simulink model "simplequeu"  (R2013a)
settings: Solver=ode45  StartTime=0.0  StopTime=10.0  RelTol=1e-3
undefined symbols (not defined in the file or in its folder): des, gcbh
settings Model: Creator=daniel  LastModifiedBy=daniel

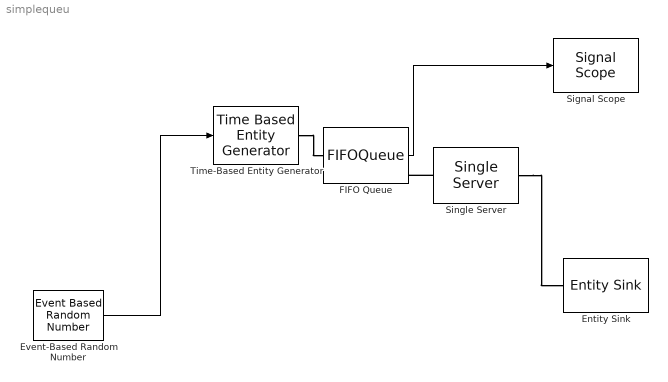
== system simplequeu ==
  Entity Sink : EntitySink  StatNumberArrived=on
  Event-Based Random Number : EventBasedRandomNumber  Distribution=Gaussian (normal)  meanNorm=90  stdNorm=3
  FIFO Queue : FIFOQueue  Capacity=250  StatNumberInBlock=on  StatAverageWait=on
      settings: OutputPortMap=o1,o2
  Signal Scope : SignalScope  LoadFcn=des.scope.CallbackSupport('seLoadFcn',gcbh)  StartFcn=des.scope.CallbackSupport('seStartFcn',gcbh)  StopFcn=des.scope.CallbackSupport('seStopFcn',gcbh)
      settings: CopyFcn=des.scope.CallbackSupport('seCopyFcn',gcbh)  DeleteFcn=des.scope.CallbackSupport('seDeleteFcn',gcbh)  PreSaveFcn=des.scope.CallbackSupport('sePreSaveFcn',gcbh)  NameChangeFcn=des.scope.CallbackSupport('seNameChangeFcn',gcbh)  OpenFcn=des.scope.CallbackSupport('seOpenFcn',gcbh)
  Single Server : SingleServer
  Time-Based Entity Generator : TimeBasedEntityGenerator  GenerateEntitiesUpon=Intergeneration time from port t  Distribution=Exponential  PriorityEntityGeneration=9
  wires:
  FIFO Queue/2 -> Signal Scope/1
  Event-Based Random Number/1 -> Time-Based Entity Generator/1
  connections:
  Single Server/LConn1 -- FIFO Queue/RConn1
  Time-Based Entity Generator/RConn1 -- FIFO Queue/LConn1
  Single Server/RConn1 -- Entity Sink/LConn1
